simulink model "machWorksSim"  (R2025b)
settings: Solver=ode4  StartTime=0.0  StopTime=100  FixedStep=0.01  RelTol=1e-3
libraries: simulink x1
settings Model: Creator=willf  LastModifiedBy=willf

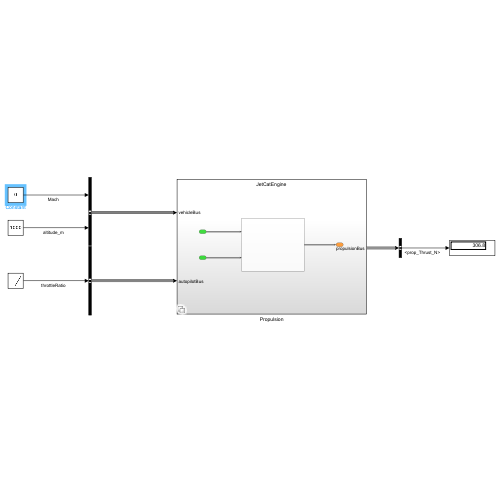
[thumbnail: Simulink's stored preview of the top-level diagram]
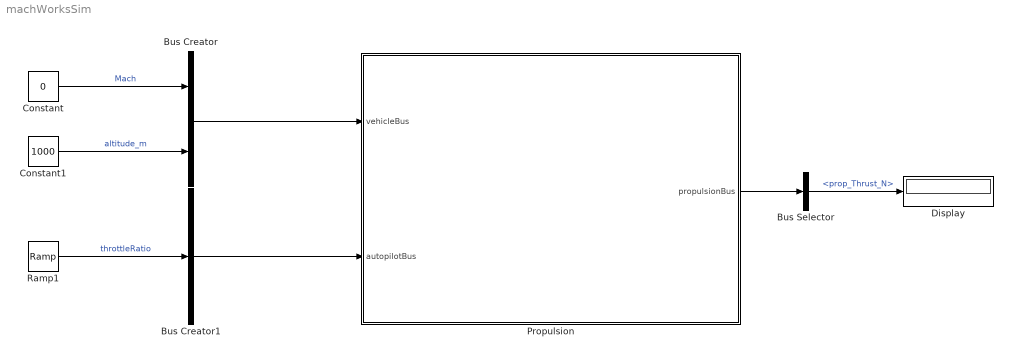
== system machWorksSim ==
  Bus Creator : BusCreator  Inputs=2
  Bus Creator1 : BusCreator  Inputs=1
  Bus Selector : BusSelector  OutputSignals=prop_Thrust_N
  Constant : Constant  Value=0
  Constant1 : Constant  Value=1000
  Display : Display
  Propulsion : Subsystem  Variant=on
  Ramp1 : simulink/Sources/Ramp  slope=1/100  start=0  InitialOutput=0
  wires:
  Bus Creator/1 -> Propulsion/1(vehicleBus)
  Constant1/1 -> Bus Creator/2  "altitude_m"
  Constant/1 -> Bus Creator/1  "Mach"
  Bus Creator1/1 -> Propulsion/2(autopilotBus)
  Ramp1/1 -> Bus Creator1/1  "throttleRatio"
  Propulsion/1(propulsionBus) -> Bus Selector/1
  Bus Selector/1 -> Display/1  "<prop_Thrust_N>"

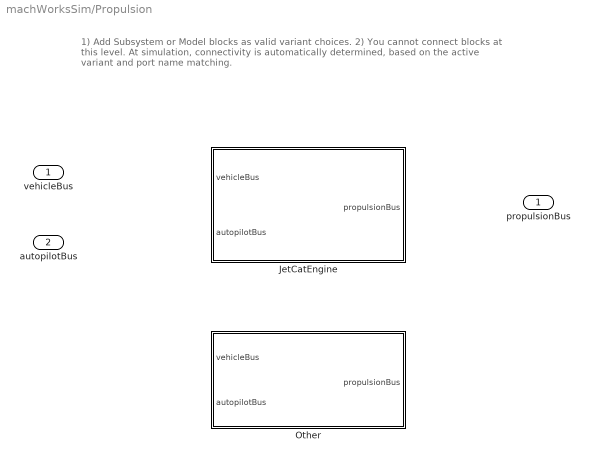
== system machWorksSim/Propulsion ==
  note: 1) Add Subsystem or Model blocks as valid variant choices.
      | 2) You cannot connect blocks at this level. At simulation, connectivity is automatically
      | determined, based on the active variant and port name matching.
  vehicleBus : Inport
  autopilotBus : Inport  Port=2
  JetCatEngine : Subsystem  VariantControl=true
  Other : Subsystem  VariantControl=false
  propulsionBus : Outport

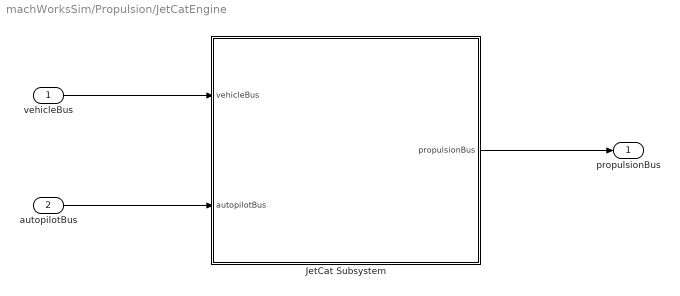
== system machWorksSim/Propulsion/JetCatEngine ==
  vehicleBus : Inport
  autopilotBus : Inport  Port=2
  JetCat Subsystem : Subsystem  Variant=on
  propulsionBus : Outport
  wires:
  vehicleBus/1 -> JetCat Subsystem/1(vehicleBus)
  autopilotBus/1 -> JetCat Subsystem/2(autopilotBus)
  JetCat Subsystem/1(propulsionBus) -> propulsionBus/1

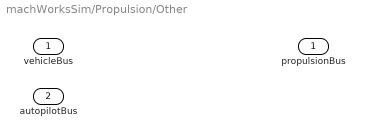
== system machWorksSim/Propulsion/Other ==
  vehicleBus : Inport
  autopilotBus : Inport  Port=2
  propulsionBus : Outport

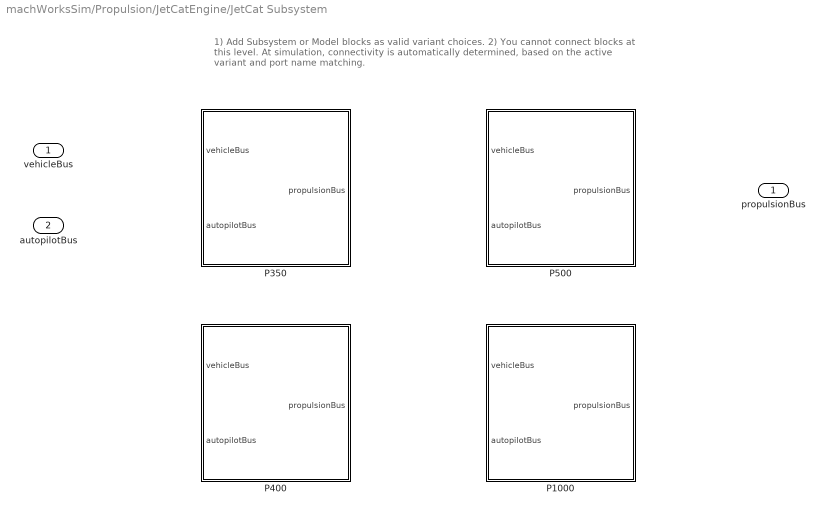
== system machWorksSim/Propulsion/JetCatEngine/JetCat Subsystem ==
  note: 1) Add Subsystem or Model blocks as valid variant choices.
      | 2) You cannot connect blocks at this level. At simulation, connectivity is automatically
      | determined, based on the active variant and port name matching.
  vehicleBus : Inport
  autopilotBus : Inport  Port=2
  P1000 : Subsystem  TreatAsAtomicUnit=on  VariantControl=false
  P350 : Subsystem  TreatAsAtomicUnit=on  VariantControl=true
  P400 : Subsystem  TreatAsAtomicUnit=on  VariantControl=false
  P500 : Subsystem  TreatAsAtomicUnit=on  VariantControl=false
  propulsionBus : Outport

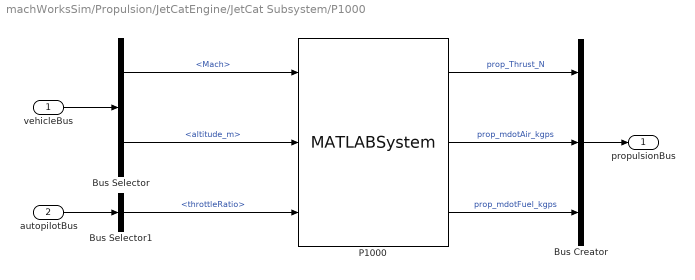
== system machWorksSim/Propulsion/JetCatEngine/JetCat Subsystem/P1000 ==
  vehicleBus : Inport
  autopilotBus : Inport  Port=2
  Bus Creator : BusCreator  Inputs=3
  Bus Selector : BusSelector  OutputSignals=Mach,altitude_m
  Bus Selector1 : BusSelector  OutputSignals=throttleRatio
  P1000 : MATLABSystem  System=P1000  PressureRatio=4  AirMassFlowMax=1.8  FuelConsumptionMax=0.00064766666666666662  FuelConsumptionMin=0.0012283333333333334  Mass=11  MinRPM=19000  MaxRPM=615000  MinThrust=45  MaxThrust=11000  SFC=0.127  Pi_d=0.95
      mask Type: P1000
  propulsionBus : Outport
  wires:
  vehicleBus/1 -> Bus Selector/1
  Bus Selector/1 -> P1000/1  "<Mach>"
  Bus Selector/2 -> P1000/2  "<altitude_m>"
  autopilotBus/1 -> Bus Selector1/1
  Bus Selector1/1 -> P1000/3  "<throttleRatio>"
  Bus Creator/1 -> propulsionBus/1
  P1000/2 -> Bus Creator/2  "prop_mdotAir_kgps"
  P1000/3 -> Bus Creator/3  "prop_mdotFuel_kgps"
  P1000/1 -> Bus Creator/1  "prop_Thrust_N"

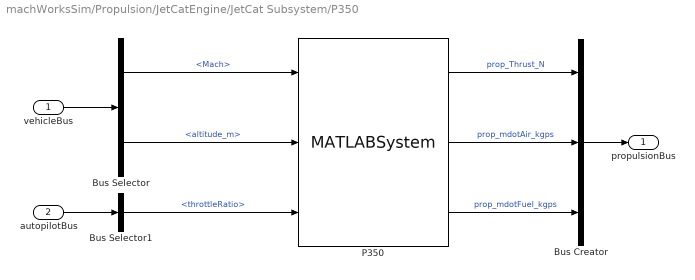
== system machWorksSim/Propulsion/JetCatEngine/JetCat Subsystem/P350 ==
  vehicleBus : Inport
  autopilotBus : Inport  Port=2
  Bus Creator : BusCreator  Inputs=3
  Bus Selector : BusSelector  OutputSignals=Mach,altitude_m
  Bus Selector1 : BusSelector  OutputSignals=throttleRatio
  P350 : MATLABSystem  System=P350  PressureRatio=3.8  AirMassFlowMax=0.65  FuelConsumptionMax=0.00026465000000000006  FuelConsumptionMin=3.3053333333333331e-05  Mass=2.89  MinRPM=30000  MaxRPM=105000  MinThrust=15.5  MaxThrust=360  SFC=0.158  Pi_d=0.95
      mask Type: P350
  propulsionBus : Outport
  wires:
  vehicleBus/1 -> Bus Selector/1
  Bus Selector/1 -> P350/1  "<Mach>"
  Bus Selector/2 -> P350/2  "<altitude_m>"
  autopilotBus/1 -> Bus Selector1/1
  Bus Selector1/1 -> P350/3  "<throttleRatio>"
  P350/2 -> Bus Creator/2  "prop_mdotAir_kgps"
  P350/1 -> Bus Creator/1  "prop_Thrust_N"
  P350/3 -> Bus Creator/3  "prop_mdotFuel_kgps"
  Bus Creator/1 -> propulsionBus/1

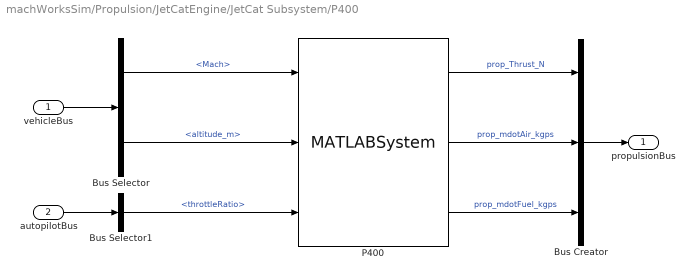
== system machWorksSim/Propulsion/JetCatEngine/JetCat Subsystem/P400 ==
  vehicleBus : Inport
  autopilotBus : Inport  Port=2
  Bus Creator : BusCreator  Inputs=3
  Bus Selector : BusSelector  OutputSignals=Mach,altitude_m
  Bus Selector1 : BusSelector  OutputSignals=throttleRatio
  P400 : MATLABSystem  System=P400  PressureRatio=3.8  AirMassFlowMax=0.67  FuelConsumptionMax=0.00031088  FuelConsumptionMin=4.4666666666666677e-05  Mass=4.01  MinRPM=30000  MaxRPM=98000  MinThrust=14  MaxThrust=425  SFC=0.157  Pi_d=0.95
      mask Type: P400
  propulsionBus : Outport
  wires:
  vehicleBus/1 -> Bus Selector/1
  Bus Selector/1 -> P400/1  "<Mach>"
  Bus Selector/2 -> P400/2  "<altitude_m>"
  autopilotBus/1 -> Bus Selector1/1
  Bus Selector1/1 -> P400/3  "<throttleRatio>"
  Bus Creator/1 -> propulsionBus/1
  P400/2 -> Bus Creator/2  "prop_mdotAir_kgps"
  P400/3 -> Bus Creator/3  "prop_mdotFuel_kgps"
  P400/1 -> Bus Creator/1  "prop_Thrust_N"

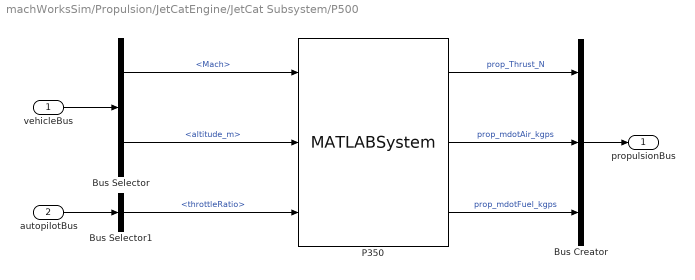
== system machWorksSim/Propulsion/JetCatEngine/JetCat Subsystem/P500 ==
  vehicleBus : Inport
  autopilotBus : Inport  Port=2
  Bus Creator : BusCreator  Inputs=3
  Bus Selector : BusSelector  OutputSignals=Mach,altitude_m
  Bus Selector1 : BusSelector  OutputSignals=throttleRatio
  P350 : MATLABSystem  System=P500  PressureRatio=3.6  AirMassFlowMax=0.9  FuelConsumptionMax=0.00034616666666666671  FuelConsumptionMin=6.7e-05  Mass=5.4  MinRPM=26000  MaxRPM=80000  MinThrust=28  MaxThrust=492  SFC=0.151  Pi_d=0.95
      mask Type: P500
  propulsionBus : Outport
  wires:
  vehicleBus/1 -> Bus Selector/1
  Bus Selector/1 -> P350/1  "<Mach>"
  Bus Selector/2 -> P350/2  "<altitude_m>"
  autopilotBus/1 -> Bus Selector1/1
  Bus Selector1/1 -> P350/3  "<throttleRatio>"
  Bus Creator/1 -> propulsionBus/1
  P350/2 -> Bus Creator/2  "prop_mdotAir_kgps"
  P350/3 -> Bus Creator/3  "prop_mdotFuel_kgps"
  P350/1 -> Bus Creator/1  "prop_Thrust_N"
